simulink model "thermal_zones"  (R2017a)
settings: Solver=VariableStepAuto  StartTime=0.0  StopTime=50000  RelTol=1e-3
settings Model: Creator=info  LastModifiedBy=info

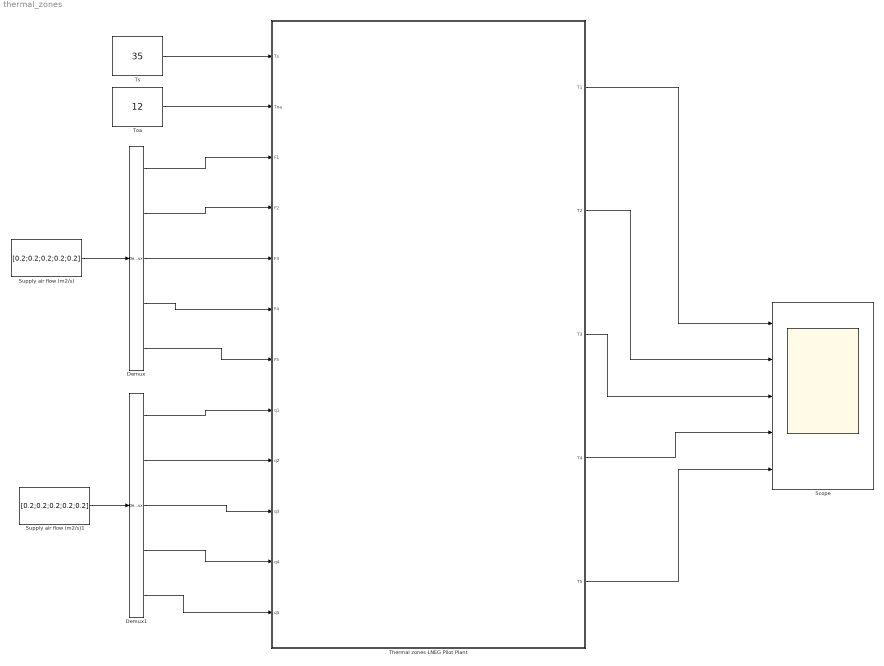
== system thermal_zones ==
  Demux : Demux  Outputs=5
  Demux1 : Demux  Outputs=5
  Scope : Scope  NumInputPorts=5
  Supply air flow (m2/s) : Constant  Value=[0.2;0.2;0.2;0.2;0.2]
  Supply air flow (m2/s)1 : Constant  Value=[0.2;0.2;0.2;0.2;0.2]
  Thermal zones LNEG Pilot Plant : Subsystem
      mask Display: image('building.PNG');
  Toa : Constant  Value=12
  Ts : Constant  Value=35
  wires:
  Ts/1 -> Thermal zones LNEG Pilot Plant/1("Ts ")
  Toa/1 -> Thermal zones LNEG Pilot Plant/2(Toa)
  Demux/5 -> Thermal zones LNEG Pilot Plant/7(F5)
  Demux/1 -> Thermal zones LNEG Pilot Plant/3("F1 ")
  Demux/2 -> Thermal zones LNEG Pilot Plant/4(F2)
  Demux/3 -> Thermal zones LNEG Pilot Plant/5(F3)
  Demux/4 -> Thermal zones LNEG Pilot Plant/6(F4)
  Supply air flow (m2/s)/1 -> Demux/1
  Demux1/2 -> Thermal zones LNEG Pilot Plant/9(q2)
  Demux1/1 -> Thermal zones LNEG Pilot Plant/8(q1)
  Demux1/3 -> Thermal zones LNEG Pilot Plant/10(q3)
  Demux1/4 -> Thermal zones LNEG Pilot Plant/11(q4)
  Demux1/5 -> Thermal zones LNEG Pilot Plant/12(q5)
  Supply air flow (m2/s)1/1 -> Demux1/1
  Thermal zones LNEG Pilot Plant/1(T1) -> Scope/1
  Thermal zones LNEG Pilot Plant/2(T2) -> Scope/2
  Thermal zones LNEG Pilot Plant/3(T3) -> Scope/3
  Thermal zones LNEG Pilot Plant/4(T4) -> Scope/4
  Thermal zones LNEG Pilot Plant/5(T5) -> Scope/5

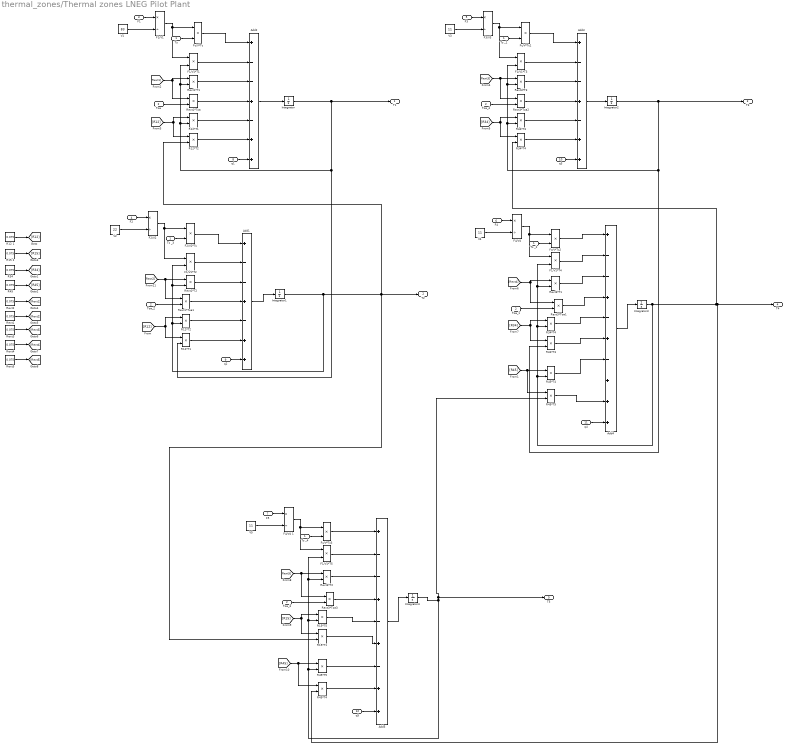
== system thermal_zones/Thermal zones LNEG Pilot Plant ==
  "Ts " : Inport
  Toa : Inport  Port=2
  "F1 " : Inport  Port=3
  F2 : Inport  Port=4
  F3 : Inport  Port=5
  F4 : Inport  Port=6
  F5 : Inport  Port=7
  q1 : Inport  Port=8
  q2 : Inport  Port=9
  q3 : Inport  Port=10
  q4 : Inport  Port=11
  q5 : Inport  Port=12
  Add1 : Sum  Inputs=+--+-++
  Add2 : Sum  Inputs=+--+-++
  Add3 : Sum  Inputs=+--+-++
  Add4 : Sum  Inputs=+--+-+-+++
  Add5 : Sum  Inputs=+--+-+-++
  F1/V1 : Product  Inputs=*/
  F1/V1*T{1..5} (5 alike) : Product  Inputs=**
  F2/V2 : Product  Inputs=*/
  F2/V2*Ts : Product  Inputs=**
  F3/V3 : Product  Inputs=*/
  "F4/V4 " : Product  Inputs=*/
  F4/V4 1 : Product  Inputs=*/
  Fc/V*Tc{,1..3} (4 alike) : Product  Inputs=**
  Integrator{,1..4} (5 alike) : Integrator  InitialCondition=16.87
  R12 1 : Constant  Value=0.075
  R12*T1 : Product  Inputs=**
  "R12*T1 " : Product  Inputs=**
  R12*T2 : Product  Inputs=**
  "R12*T2 " : Product  Inputs=**
  R15 2 : Constant  Value=0.075
  R15*T1 : Product  Inputs=**
  R15*T5 : Product  Inputs=**
  "R34 " : Constant  Value=0.075
  R34*T3 : Product  Inputs=**
  "R34*T3  " : Product  Inputs=**
  R34*T4 : Product  Inputs=**
  "R34*T4   " : Product  Inputs=**
  "R45 " : Constant  Value=0.075
  R45*T4 : Product  Inputs=**
  "R45*T4      " : Product  Inputs=**
  R45*T5 : Product  Inputs=**
  "R45*T5    " : Product  Inputs=**
  Rext{1..5} (5 alike) : Constant  Value=0.075
  Rext1*T1 : Product  Inputs=**
  Rext1*T2 : Product  Inputs=**
  Rext1*Toa : Product  Inputs=**
  Rext1*Toa1 : Product  Inputs=**
  Rext3*T1 : Product  Inputs=**
  Rext3*T2 : Product  Inputs=**
  Rext3*T3 : Product  Inputs=**
  Rext3*Toa1 : Product  Inputs=**
  Rext3*Toa2 : Product  Inputs=**
  Rext3*Toa3 : Product  Inputs=**
  Toa_{1..4} (4 alike) : InportShadow  Port=2
  Ts _{1..4} (4 alike) : InportShadow
  V1 : Constant  Value=83
  V2 : Constant  Value=22
  V3 : Constant  Value=11
  V4 : Constant  Value=11
  V5 : Constant  Value=11
  T1 : Outport
  T2 : Outport  Port=2
  T3 : Outport  Port=3
  T4 : Outport  Port=4
  T5 : Outport  Port=5
  wires:
  Add3/1 -> Integrator2/1
  Ts _1/1 -> Fc/V*Tc1/2
  Toa_4/1 -> Rext3*Toa2/2
  R34*T4/1 -> Add3/6
  V3/1 -> F3/V3/2
  Fc/V*Tc1/1 -> Add3/1
  Rext3*T3/1 -> Add3/3
  F1/V1*T3/1 -> Add3/2
  Rext3*Toa2/1 -> Add3/4
  Integrator2/1 -> T3/1, "R34*T3  "/2, R34*T3/2, Rext3*T3/2, F1/V1*T3/2
  F3/1 -> F3/V3/1
  q3/1 -> Add3/7
  R34*T3/1 -> Add3/5
  [R34] -> R34*T4/1, R34*T3/1
  F3/V3/1 -> F1/V1*T3/1, Fc/V*Tc1/1
  [Rext3] -> Rext3*Toa2/1, Rext3*T3/1
  q5/1 -> Add5/9
  R12 1/1 -> [R12]
  Rext3*T2/1 -> Add5/3
  R15*T5/1 -> Add5/5
  R15*T1/1 -> Add5/6
  R45*T5/1 -> Add5/7
  Ts _4/1 -> Fc/V*Tc3/2
  [R45] -> R45*T4/1, R45*T5/1
  Rext3*Toa3/1 -> Add5/4
  F4/V4 1/1 -> F1/V1*T5/1, Fc/V*Tc3/1
  Add5/1 -> Integrator4/1
  Toa_3/1 -> Rext3*Toa3/2
  V5/1 -> F4/V4 1/2
  F1/V1*T5/1 -> Add5/2
  F5/1 -> F4/V4 1/1
  [R15] -> R15*T1/1, R15*T5/1
  [Rext5] -> Rext3*Toa3/1, Rext3*T2/1
  Fc/V*Tc3/1 -> Add5/1
  R15 2/1 -> [R15]
  Rext2/1 -> [Rext1]
  Rext3/1 -> [Rext3]
  Rext1/1 -> [Rext2]
  Rext4/1 -> [Rext4]
  Rext5/1 -> [Rext5]
  [R45] -> "R45*T5    "/1, "R45*T4      "/1
  "R45*T4      "/1 -> Add4/7
  Toa/1 -> Rext1*Toa/2
  q1/1 -> Add2/7
  Integrator/1 -> T1/1, "R12*T1 "/2, R12*T1/2, Rext1*T1/2, F1/V1*T1/2
  F1/V1/1 -> F1/V1*T1/1, Fc/V*Tc/1
  V1/1 -> F1/V1/2
  Add2/1 -> Integrator/1
  "F1 "/1 -> F1/V1/1
  Fc/V*Tc/1 -> Add2/1
  F1/V1*T1/1 -> Add2/2
  "Ts "/1 -> Fc/V*Tc/2
  R12*T1/1 -> Add2/5
  R12*T2/1 -> Add2/6
  [R12] -> R12*T2/1, R12*T1/1
  Rext1*Toa/1 -> Add2/4
  V2/1 -> F2/V2/2
  Toa_2/1 -> Rext1*Toa1/2
  F2/V2*Ts/1 -> Add1/1
  Rext1*Toa1/1 -> Add1/4
  q2/1 -> Add1/7
  F2/V2/1 -> F1/V1*T2/1, F2/V2*Ts/1
  Ts _3/1 -> F2/V2*Ts/2
  [R12] -> "R12*T1 "/1, "R12*T2 "/1
  Integrator1/1 -> T2/1, R15*T1/2, R12*T2/2, "R12*T2 "/2, Rext1*T2/2, F1/V1*T2/2
  Rext1*T2/1 -> Add1/3
  [Rext2] -> Rext1*Toa1/1, Rext1*T2/1
  "R12*T2 "/1 -> Add1/5
  "R12*T1 "/1 -> Add1/6
  F2/1 -> F2/V2/1
  Add1/1 -> Integrator1/1
  Rext1*T1/1 -> Add2/3
  F1/V1*T2/1 -> Add1/2
  [Rext1] -> Rext1*Toa/1, Rext1*T1/1
  "R45*T5    "/1 -> Add4/9
  R45*T4/1 -> Add5/8
  Integrator4/1 -> "R45*T5    "/2, T5/1, R45*T5/2, R15*T5/2, Rext3*T2/2, F1/V1*T5/2
  q4/1 -> Add4/10
  Integrator3/1 -> R34*T4/2, T4/1, R45*T4/2, "R45*T4      "/2, "R34*T4   "/2, Rext3*T1/2, F1/V1*T4/2
  F1/V1*T4/1 -> Add4/2
  Rext3*T1/1 -> Add4/3
  V4/1 -> "F4/V4 "/2
  Fc/V*Tc2/1 -> Add4/1
  "R34*T4   "/1 -> Add4/5
  Rext3*Toa1/1 -> Add4/4
  Add4/1 -> Integrator3/1
  F4/1 -> "F4/V4 "/1
  Toa_1/1 -> Rext3*Toa1/2
  [R34] -> "R34*T3  "/1, "R34*T4   "/1
  "R34*T3  "/1 -> Add4/6
  "F4/V4 "/1 -> F1/V1*T4/1, Fc/V*Tc2/1
  Ts _2/1 -> Fc/V*Tc2/2
  [Rext4] -> Rext3*Toa1/1, Rext3*T1/1
  "R45 "/1 -> [R45]
  "R34 "/1 -> [R34]
